simulink model "Filtering"  (R2018a)
settings: Solver=VariableStepAuto  StartTime=0.0  StopTime=10.0  RelTol=1e-3
values from neighbouring files (symbols this model uses):
  T = 1/Fs    (= 5e-05)    [SimVar.m]
undefined symbols (not defined in the file or in its folder): G
libraries: dspsrcs4 x7, dspfdesign x1
settings Model: Creator=Daniel  LastModifiedBy=Daniel

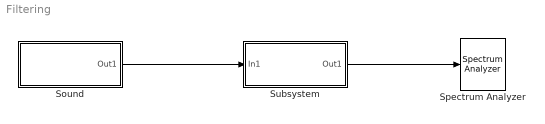
== system Filtering ==
  "Sound " : Subsystem
  Spectrum Analyzer : SpectrumAnalyzer
  Subsystem : Subsystem
  wires:
  Subsystem/1(Out1) -> Spectrum Analyzer/1
  "Sound "/1(Out1) -> Subsystem/1(In1)

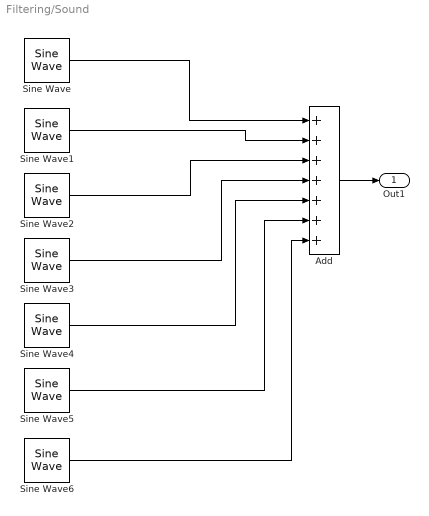
== system Filtering/Sound  ==
  Add : Sum  Inputs=+++++++
  Sine Wave : dspsrcs4/Sine Wave  Amplitude=1  Frequency=200  Phase=0  SampleMode=Discrete  OutComplex=Real  CompMethod=Trigonometric fcn  TableSize=Speed  SampleTime=T  SamplesPerFrame=1  ResetState=Restart at time zero  OutputFrames=off  dataType=double  wordLen=16  udDataType=sfix(16)  fracBitsMode=Best precision  numFracBits=15  OutDataTypeStr=double  LastOutDataTypeStr=double
  Sine Wave1 : dspsrcs4/Sine Wave  Amplitude=1  Frequency=400  Phase=0  SampleMode=Discrete  OutComplex=Real  CompMethod=Trigonometric fcn  TableSize=Speed  SampleTime=T  SamplesPerFrame=1  ResetState=Restart at time zero  OutputFrames=off  dataType=double  wordLen=16  udDataType=sfix(16)  fracBitsMode=Best precision  numFracBits=15  OutDataTypeStr=double  LastOutDataTypeStr=double
  Sine Wave2 : dspsrcs4/Sine Wave  Amplitude=1  Frequency=800  Phase=0  SampleMode=Discrete  OutComplex=Real  CompMethod=Trigonometric fcn  TableSize=Speed  SampleTime=T  SamplesPerFrame=1  ResetState=Restart at time zero  OutputFrames=off  dataType=double  wordLen=16  udDataType=sfix(16)  fracBitsMode=Best precision  numFracBits=15  OutDataTypeStr=double  LastOutDataTypeStr=double
  Sine Wave3 : dspsrcs4/Sine Wave  Amplitude=1  Frequency=1600  Phase=0  SampleMode=Discrete  OutComplex=Real  CompMethod=Trigonometric fcn  TableSize=Speed  SampleTime=T  SamplesPerFrame=1  ResetState=Restart at time zero  OutputFrames=off  dataType=double  wordLen=16  udDataType=sfix(16)  fracBitsMode=Best precision  numFracBits=15  OutDataTypeStr=double  LastOutDataTypeStr=double
  Sine Wave4 : dspsrcs4/Sine Wave  Amplitude=1  Frequency=3200  Phase=0  SampleMode=Discrete  OutComplex=Real  CompMethod=Trigonometric fcn  TableSize=Speed  SampleTime=T  SamplesPerFrame=1  ResetState=Restart at time zero  OutputFrames=off  dataType=double  wordLen=16  udDataType=sfix(16)  fracBitsMode=Best precision  numFracBits=15  OutDataTypeStr=double  LastOutDataTypeStr=double
  Sine Wave5 : dspsrcs4/Sine Wave  Amplitude=1  Frequency=6400  Phase=0  SampleMode=Discrete  OutComplex=Real  CompMethod=Trigonometric fcn  TableSize=Speed  SampleTime=T  SamplesPerFrame=1  ResetState=Restart at time zero  OutputFrames=off  dataType=double  wordLen=16  udDataType=sfix(16)  fracBitsMode=Best precision  numFracBits=15  OutDataTypeStr=double  LastOutDataTypeStr=double
  Sine Wave6 : dspsrcs4/Sine Wave  Amplitude=1  Frequency=8000  Phase=0  SampleMode=Discrete  OutComplex=Real  CompMethod=Trigonometric fcn  TableSize=Speed  SampleTime=T  SamplesPerFrame=1  ResetState=Restart at time zero  OutputFrames=off  dataType=double  wordLen=16  udDataType=sfix(16)  fracBitsMode=Best precision  numFracBits=15  OutDataTypeStr=double  LastOutDataTypeStr=double
  Out1 : Outport
  wires:
  Sine Wave/1 -> Add/1
  Sine Wave1/1 -> Add/2
  Sine Wave2/1 -> Add/3
  Sine Wave3/1 -> Add/4
  Sine Wave4/1 -> Add/5
  Sine Wave5/1 -> Add/6
  Sine Wave6/1 -> Add/7
  Add/1 -> Out1/1

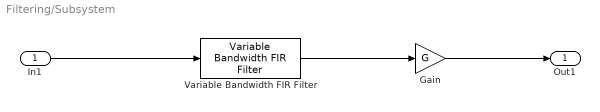
== system Filtering/Subsystem ==
  In1 : Inport  OutDataTypeStr=double
  Gain : Gain  Gain=G
  Variable Bandwidth FIR Filter : dspfdesign/Variable Bandwidth FIR Filter  FilterOrder=30  FilterType=Bandpass  CutoffFrequencyPort=off  CutoffFrequency=512  CenterFrequencyPort=off  CenterFrequency=3500  BandwidthPort=off  Bandwidth=1000  Window=Hamming  KaiserWindowParameter=.5  SidelobeAttenuation=60  InheritSampleRate=off  SampleRate=Fs  SimulateUsing=Code generation
      settings: SourceProductName=DSP System Toolbox  SourceProductBaseCode=DS
  Out1 : Outport
  wires:
  In1/1 -> Variable Bandwidth FIR Filter/1
  Gain/1 -> Out1/1
  Variable Bandwidth FIR Filter/1 -> Gain/1
